simulink model "CTC_test"  (Simulink 7.4)
settings: Solver=FixedStepDiscrete  StartTime=0.0  StopTime=inf  FixedStep=0.01  RelTol=1e-3
libraries: CTC_lib x1, simulink x1
Description:
  | $Author:Zhao XiangRi$
  | $Date:2015/03/26$
  | $Revision:1.0$
settings Model: Creator=zhaoxiangri  LastModifiedBy=zhaoxiangri  BufferReuse=off
settings DataIOCC: SaveFormat=Structure  SaveOutput=off  SaveTime=off
settings OptimizationCC: BlockReduction=off  OptimizeBlockIOStorage=off  BufferReuse=off  ExpressionFolding=off  ExpressionDepthLimit=128  LocalBlockOutputs=off  StateBitsets=on  DataBitsets=on  UseTempVars=on  EfficientFloat2IntCast=on  OptimizeModelRefInitCode=on  LifeSpan=Inf
settings DebuggingCC: RTPrefix=none  SignalInfNanChecking=warning  SignalResolutionControl=TryResolveAll  MultiTaskDSMMsg=none  MultiTaskCondExecSysMsg=warning  MultiTaskRateTransMsg=warning  IntegerOverflowMsg=error  ParameterDowncastMsg=none  ParameterPrecisionLossMsg=none  UnnecessaryDatatypeConvMsg=warning  InvalidFcnCallConnMsg=warning  FcnCallInpInsideContextMsg=Enable All  UnconnectedInputMsg=error  UnconnectedOutputMsg=error  UnconnectedLineMsg=error  UniqueDataStoreMsg=warning  RootOutportRequireBusObject=none  ModelReferenceIOMsg=warning  ModelReferenceVersionMismatchMessage=warning  ModelReferenceIOMismatchMessage=warning  ModelReferenceCSMismatchMessage=warning  StrictBusMsg=ErrorLevel1
settings HardwareCC: ProdIntDivRoundTo=Zero  ProdEndianess=BigEndian  ProdHWDeviceType=Freescale->32-bit PowerPC
settings RTWCC: SystemTargetFile=ert.tlc  GenCodeOnly=on  TemplateMakefile=ert_default_tmf  Description=Real-Time Workshop Embedded Coder  GenerateReport=on  RTWVerbose=off  ProcessScript=ert_make_rtw_hook  IncludeHyperlinkInReport=on  LaunchReport=on
settings CodeAppCC: ForceParamTrailComments=on  IgnoreCustomStorageClasses=off
settings ERTTargetCC: MultiwordLength=2048  GenerateSampleERTMain=on  ERTCustomFileTemplate=example_file_process.tlc  ConvertIfToSwitch=off

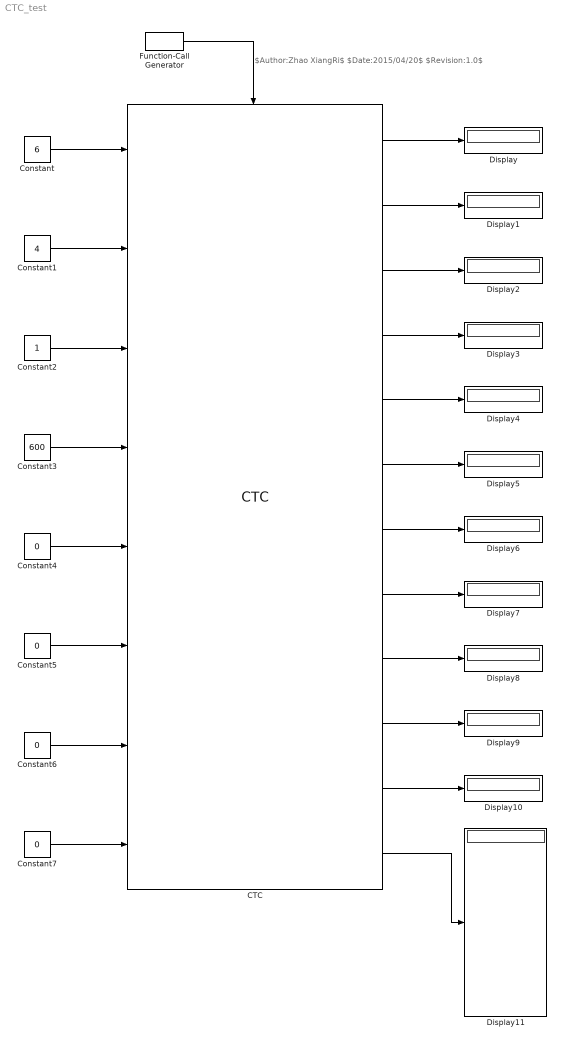
== system CTC_test ==
  note: $Author:Zhao XiangRi$
      | $Date:2015/04/20$
      | $Revision:1.0$
  CTC : CTC_lib/CTC  Description=|  SystemSampleTime=-1
      | $Author:Zhao XiangRi$
      | $Date:2015/03/26$    
      | $Revision:1.0$
  Constant : Constant  Value=6  OutDataTypeMode=uint8  OutDataType=fixdt(1, 16)  OutScaling=2^0  OutDataTypeStr=uint8
  Constant1 : Constant  Value=4  OutDataTypeMode=uint8  OutDataType=fixdt(1, 16)  OutScaling=2^0  OutDataTypeStr=uint8
  Constant2 : Constant  OutDataTypeMode=uint8  OutDataType=fixdt(1, 16)  OutScaling=2^0  OutDataTypeStr=uint8
  Constant3 : Constant  Value=600  OutDataTypeMode=single  OutDataType=fixdt(1, 16)  OutScaling=2^0  OutDataTypeStr=single
  Constant4 : Constant  Value=0  OutDataTypeMode=single  OutDataType=fixdt(1, 16)  OutScaling=2^0  OutDataTypeStr=single
  Constant5 : Constant  Value=0  OutDataTypeMode=single  OutDataType=fixdt(1, 16)  OutScaling=2^0  OutDataTypeStr=single
  Constant6 : Constant  Value=0  OutDataType=fixdt(1, 16)  OutScaling=2^0
  Constant7 : Constant  Value=0  OutDataTypeMode=single  OutDataType=fixdt(1, 16)  OutScaling=2^0  OutDataTypeStr=single
  Display{,1..11} (12 alike) : Display
  Function-Call Generator : simulink/Ports & Subsystems/Function-Call Generator  sample_time=1  numberOfIterations=1
  wires:
  Function-Call Generator/1 -> CTC/Trigger
  CTC/1 -> Display/1
  CTC/2 -> Display1/1
  CTC/3 -> Display2/1
  CTC/4 -> Display3/1
  CTC/5 -> Display4/1
  CTC/6 -> Display5/1
  CTC/7 -> Display6/1
  CTC/8 -> Display7/1
  CTC/9 -> Display8/1
  CTC/10 -> Display9/1
  CTC/11 -> Display10/1
  Constant/1 -> CTC/1
  Constant1/1 -> CTC/2
  Constant2/1 -> CTC/3
  Constant3/1 -> CTC/4
  Constant4/1 -> CTC/5
  Constant5/1 -> CTC/6
  Constant6/1 -> CTC/7
  Constant7/1 -> CTC/8
  CTC/12 -> Display11/1
